simulink model "clock_jitter"  (R2021b)
settings: Solver=VariableStepAuto  StartTime=0.0  StopTime=10.0  RelTol=1e-3
values from neighbouring files (symbols this model uses):
  bits_number = 13    [launch_pipeline_clock.m]
  fin = antismear(fin_pre,fs,nfft)    [launch_pipeline_clock.m]
  meanvalue = 0.01    [launch_pipeline_clock.m]
  ts = 1/fs    (= 1)    [launch_pipeline_clock.m]
  variance = 1e-30    [launch_pipeline_clock.m]
(part 2 of 2)

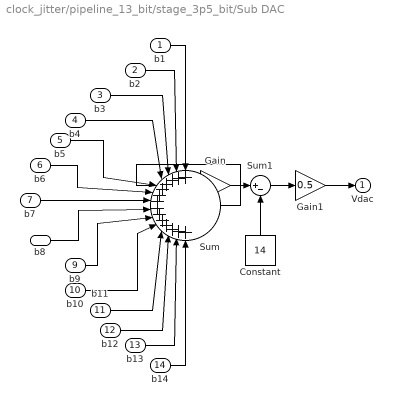
== system clock_jitter/pipeline_13_bit/stage_3p5_bit/Sub DAC ==
  b1 : Inport
  b2 : Inport  Port=2
  b3 : Inport  Port=3
  b4 : Inport  Port=4
  b5 : Inport  Port=5
  b6 : Inport  Port=6
  b7 : Inport  Port=7
  b8 : Inport  Port=8
  b9 : Inport  Port=9
  b10 : Inport  Port=10
  b11 : Inport  Port=11
  b12 : Inport  Port=12
  b13 : Inport  Port=13
  b14 : Inport  Port=14
  Constant : Constant  Value=14
  Gain : Gain  Gain=2
  Gain1 : Gain  Gain=0.5
  Sum : Sum  Inputs=++++++++++++++
  Sum1 : Sum  Inputs=|+-
  Vdac : Outport
  wires:
  b1/1 -> Sum/1
  b2/1 -> Sum/2
  b3/1 -> Sum/3
  b4/1 -> Sum/4
  b5/1 -> Sum/5
  b6/1 -> Sum/6
  Sum/1 -> Gain/1
  Gain/1 -> Sum1/1
  Constant/1 -> Sum1/2
  Sum1/1 -> Gain1/1
  Gain1/1 -> Vdac/1
  b7/1 -> Sum/7
  b8/1 -> Sum/8
  b9/1 -> Sum/9
  b10/1 -> Sum/10
  b11/1 -> Sum/11
  b12/1 -> Sum/12
  b13/1 -> Sum/13
  b14/1 -> Sum/14
